simulink model "PathPlanning"  (R2019b)
settings: Solver=VariableStepAuto  StartTime=0.0  StopTime=10.0  RelTol=1e-3
settings Model: Creator=Mouleeswar  LastModifiedBy=naika

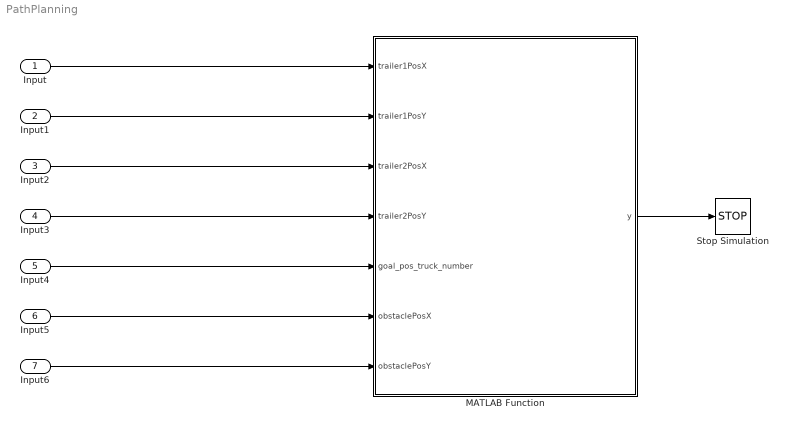
== system PathPlanning ==
  Input : Inport  OutDataTypeStr=double
  Input1 : Inport  Port=2  OutDataTypeStr=double
  Input2 : Inport  Port=3  OutDataTypeStr=double
  Input3 : Inport  Port=4  OutDataTypeStr=double
  Input4 : Inport  Port=5  OutDataTypeStr=int16
  Input5 : Inport  Port=6  OutDataTypeStr=double
  Input6 : Inport  Port=7  OutDataTypeStr=double
  MATLAB Function : MATLAB Function  TreatAsAtomicUnit=on
  Stop Simulation : Stop
  wires:
  Input4/1 -> MATLAB Function/5(goal_pos_truck_number)
  Input/1 -> MATLAB Function/1(trailer1PosX)
  Input1/1 -> MATLAB Function/2(trailer1PosY)
  Input2/1 -> MATLAB Function/3(trailer2PosX)
  Input5/1 -> MATLAB Function/6(obstaclePosX)
  Input3/1 -> MATLAB Function/4(trailer2PosY)
  Input6/1 -> MATLAB Function/7(obstaclePosY)
  MATLAB Function/1(y) -> Stop Simulation/1

== matlab function PathPlanning/MATLAB Function ==
  data: trailer1PosX input; trailer1PosY input; trailer2PosX input; trailer2PosY input; goal_pos_truck_number input; obstaclePosX input; obstaclePosY input; y output
function  y = fcn(trailer1PosX,trailer1PosY,trailer2PosX,trailer2PosY, goal_pos_truck_number, obstaclePosX,obstaclePosY)

coder.extrinsic('RRT');
y =0;

RRT(trailer1PosX,trailer1PosY,trailer2PosX,trailer2PosY, goal_pos_truck_number, obstaclePosX,obstaclePosY);
y=1;
end
